simulink model "underwater_sim_2015a"  (R2015b)
settings: Solver=ode45  StartTime=0.0  StopTime=200  RelTol=1e-3
InitFcn:
  | param
undefined symbols (not defined in the file or in its folder): AP, P, underwater_ctrl
settings Model: Creator=beard  LastModifiedBy=jae
settings DataIOCC: SaveFormat=Array  SignalLoggingSaveFormat=ModelDataLogs
settings OptimizationCC: ExpressionDepthLimit=2147483647  InitFltsAndDblsToZero=on
settings DebuggingCC: UnderspecifiedInitializationDetection=Classic  MergeDetectMultiDrivingBlocksExec=none  SolverPrmCheckMsg=warning  FcnCallInpInsideContextMsg=UseLocalSettings  StateNameClashWarn=warning
settings HardwareCC: ProdBitPerPointer=32  ProdLargestAtomicFloat=None  ProdIntDivRoundTo=Undefined  ProdEndianess=Unspecified  ProdWordSize=32  ProdHWDeviceType=32-bit Generic
settings GRTTargetCC: GeneratePreprocessorConditionals=Disable all  CombineOutputUpdateFcns=off  GRTInterface=on
settings ConfigComp: CovModelRefEnable=Off

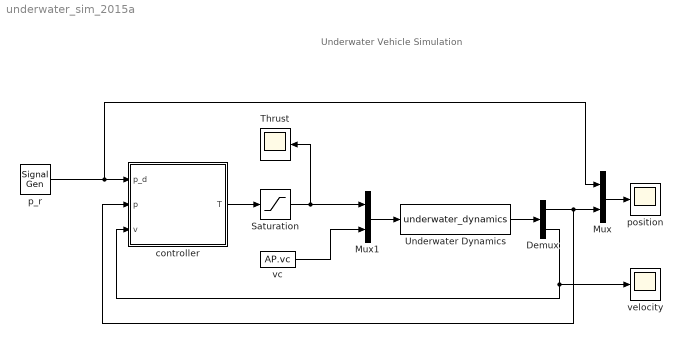
== system underwater_sim_2015a ==
  note: Underwater Vehicle Simulation
  Demux : Demux  Outputs=2
  Mux : Mux  Inputs=2
  Mux1 : Mux  Inputs=2
  Saturation : Saturate  UpperLimit=P.Tmax  LowerLimit=-P.Tmax
  Thrust : Scope
  Underwater Dynamics : S-Function  FunctionName=underwater_dynamics  Parameters=AP  SFunctionDeploymentMode=off  EnableBusSupport=off
  controller : Subsystem
  p_r : SignalGenerator  WaveForm=square  Frequency=.01
  position : Scope
  vc : Constant  Value=AP.vc
  velocity : Scope
  wires:
  Underwater Dynamics/1 -> Demux/1
  p_r/1 -> Mux/1, controller/1(p_d)
  Saturation/1 -> Thrust/1, Mux1/1
  controller/1(T) -> Saturation/1
  Demux/2 -> velocity/1, controller/3(v)
  Demux/1 -> controller/2(p), Mux/2
  Mux/1 -> position/1
  Mux1/1 -> Underwater Dynamics/1
  vc/1 -> Mux1/2

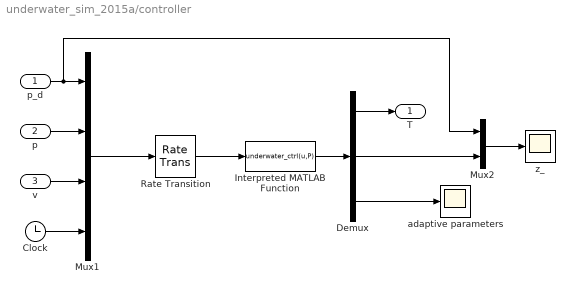
== system underwater_sim_2015a/controller ==
  p_d : Inport
  p : Inport  Port=2
  v : Inport  Port=3
  Clock : Clock
  Demux : Demux  Outputs=[1;1;P.num_adaptive_param]
  Interpreted MATLAB Function : MATLABFcn  MATLABFcn=underwater_ctrl(u,P)  OutputDimensions=2+P.num_adaptive_param
  Mux1 : Mux
  Mux2 : Mux  Inputs=2
  Rate Transition : RateTransition  OutPortSampleTime=P.Ts
  "adaptive parameters " : Scope
  z_ : Scope
  T : Outport
  wires:
  Mux1/1 -> Rate Transition/1
  Rate Transition/1 -> Interpreted MATLAB Function/1
  p/1 -> Mux1/2
  v/1 -> Mux1/3
  Clock/1 -> Mux1/4
  Interpreted MATLAB Function/1 -> Demux/1
  Demux/1 -> T/1
  Demux/2 -> Mux2/2
  Mux2/1 -> z_/1
  Demux/3 -> "adaptive parameters "/1
  p_d/1 -> Mux2/1, Mux1/1
